simulink model "telegraph"  (R2015b)
settings: Solver=FixedStepAuto  StartTime=0.0  StopTime=50  FixedStep=0.1  RelTol=1e-3
libraries: robotlib x18, dspsrcs4 x6
settings Model: Creator=erik  LastModifiedBy=rasrack
settings OptimizationCC: OptimizeModelRefInitCode=on  LifeSpan=1  MaxStackSize=64
settings HardwareCC: ProdBitPerPointer=32  ProdLargestAtomicFloat=None  ProdIntDivRoundTo=Undefined  ProdEndianess=Unspecified  ProdWordSize=32  ProdHWDeviceType=Generic->Unspecified (assume 32-bit Generic)
settings RTWCC: SystemTargetFile=ert.tlc  TemplateMakefile=ert_default_tmf  Description=Embedded Coder  Toolchain=Catkin  TargetLang=C++
settings CodeAppCC: IgnoreCustomStorageClasses=off
settings ERTTargetCC: GenerateSampleERTMain=on

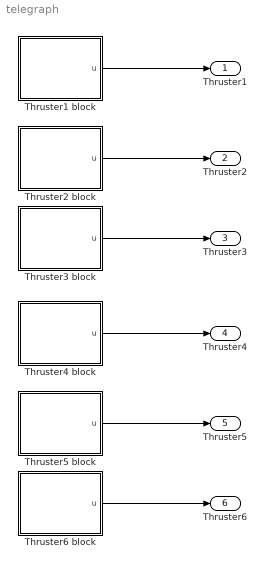
== system telegraph ==
  Thruster1 block : Subsystem
  Thruster2 block : Subsystem
  Thruster3 block : Subsystem
  Thruster4 block : Subsystem
  Thruster5 block : Subsystem
  Thruster6 block : Subsystem
  Thruster1 : Outport
  Thruster2 : Outport  Port=2
  Thruster3 : Outport  Port=3
  Thruster4 : Outport  Port=4
  Thruster5 : Outport  Port=5
  Thruster6 : Outport  Port=6
  wires:
  Thruster1 block/1(u) -> Thruster1/1
  Thruster2 block/1(u) -> Thruster2/1
  Thruster3 block/1(u) -> Thruster3/1
  Thruster4 block/1(u) -> Thruster4/1
  Thruster5 block/1("u ") -> Thruster5/1
  Thruster6 block/1(u) -> Thruster6/1

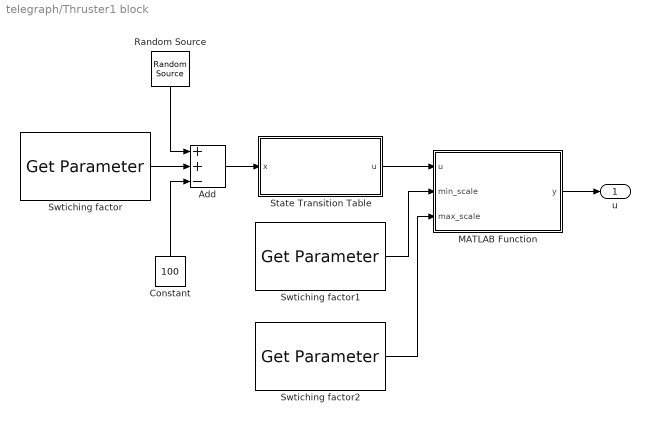
== system telegraph/Thruster1 block ==
  Add : Sum  Inputs=++-
  Constant : Constant  Value=100
  MATLAB Function : MATLAB Function  TreatAsAtomicUnit=on
  Random Source : dspsrcs4/Random Source  SrcType=Uniform  NormMethod=Ziggurat  CltLength=12  MinVal=1  MaxVal=100  MeanVal=0  VarVal=1  RepMode=Not repeatable  rawSeed=1  IsInherit=on  SampMode=Discrete  SampTime=0.1  SampFrame=1  DataType=Double  OutComplex=Real  OutputFrames=off
  State Transition Table : State Transition Table  TreatAsAtomicUnit=on
  Swtiching factor : robotlib/Get Parameter  SourceLibraryInfo=This block requires Robotics System Toolbox  ParameterSource=Specify your own  ParameterName=/matlab_controller/thruster1/switch_factor  ParameterType=int32  ParameterInitialValue=0.0  SampleTime=-1  ShowErrorCodeOutput=off  ModelName=telegraph  BlockId=ParamGet_telegraph_32
  Swtiching factor1 : robotlib/Get Parameter  SourceLibraryInfo=This block requires Robotics System Toolbox  ParameterSource=Specify your own  ParameterName=/matlab_controller/thruster1/min_scale  ParameterType=int32  ParameterInitialValue=1  SampleTime=-1  ShowErrorCodeOutput=off  ModelName=telegraph  BlockId=ParamGet_telegraph_50
  Swtiching factor2 : robotlib/Get Parameter  SourceLibraryInfo=This block requires Robotics System Toolbox  ParameterSource=Specify your own  ParameterName=/matlab_controller/thruster1/max_scale  ParameterType=int32  ParameterInitialValue=1.0  SampleTime=-1  ShowErrorCodeOutput=off  ModelName=telegraph  BlockId=ParamGet_telegraph_51
  u : Outport
  wires:
  MATLAB Function/1(y) -> u/1
  Swtiching factor1/1 -> MATLAB Function/2(min_scale)
  State Transition Table/1(u) -> MATLAB Function/1(u)
  Swtiching factor2/1 -> MATLAB Function/3(max_scale)
  Add/1 -> State Transition Table/1(x)
  Swtiching factor/1 -> Add/2
  Random Source/1 -> Add/1
  Constant/1 -> Add/3

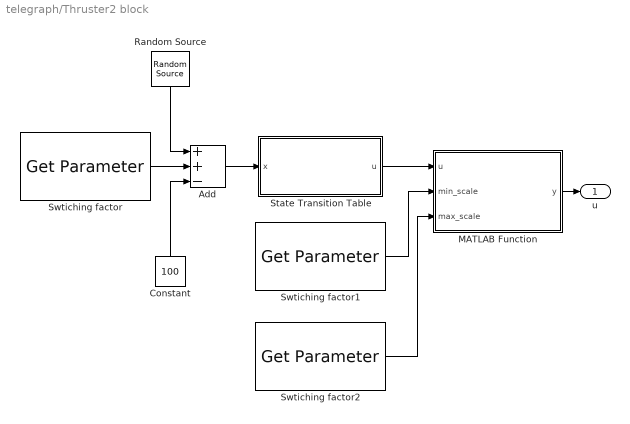
== system telegraph/Thruster2 block ==
  Add : Sum  Inputs=++-
  Constant : Constant  Value=100
  MATLAB Function : MATLAB Function  TreatAsAtomicUnit=on
  Random Source : dspsrcs4/Random Source  SrcType=Uniform  NormMethod=Ziggurat  CltLength=12  MinVal=1  MaxVal=100  MeanVal=0  VarVal=1  RepMode=Not repeatable  rawSeed=1  IsInherit=on  SampMode=Discrete  SampTime=0.1  SampFrame=1  DataType=Double  OutComplex=Real  OutputFrames=off
  State Transition Table : State Transition Table  TreatAsAtomicUnit=on
  Swtiching factor : robotlib/Get Parameter  SourceLibraryInfo=This block requires Robotics System Toolbox  ParameterSource=Specify your own  ParameterName=/matlab_controller/thruster2/switch_factor  ParameterType=int32  ParameterInitialValue=0.0  SampleTime=-1  ShowErrorCodeOutput=off  ModelName=telegraph  BlockId=ParamGet_telegraph_60
  Swtiching factor1 : robotlib/Get Parameter  SourceLibraryInfo=This block requires Robotics System Toolbox  ParameterSource=Specify your own  ParameterName=/matlab_controller/thruster2/min_scale  ParameterType=int32  ParameterInitialValue=1  SampleTime=-1  ShowErrorCodeOutput=off  ModelName=telegraph  BlockId=ParamGet_telegraph_61
  Swtiching factor2 : robotlib/Get Parameter  SourceLibraryInfo=This block requires Robotics System Toolbox  ParameterSource=Specify your own  ParameterName=/matlab_controller/thruster2/max_scale  ParameterType=int32  ParameterInitialValue=1.0  SampleTime=-1  ShowErrorCodeOutput=off  ModelName=telegraph  BlockId=ParamGet_telegraph_62
  u : Outport
  wires:
  MATLAB Function/1(y) -> u/1
  Swtiching factor1/1 -> MATLAB Function/2(min_scale)
  State Transition Table/1(u) -> MATLAB Function/1(u)
  Swtiching factor2/1 -> MATLAB Function/3(max_scale)
  Add/1 -> State Transition Table/1(x)
  Swtiching factor/1 -> Add/2
  Random Source/1 -> Add/1
  Constant/1 -> Add/3

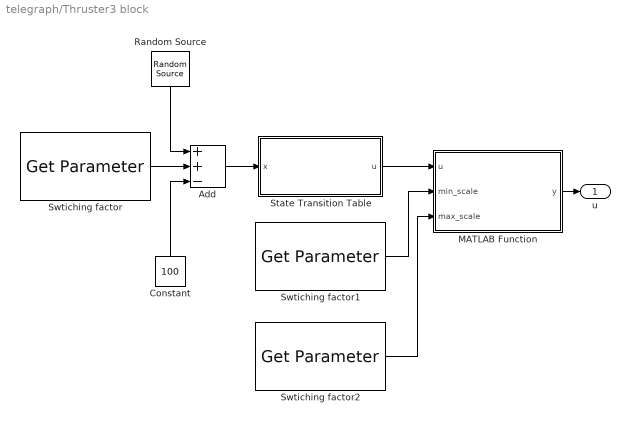
== system telegraph/Thruster3 block ==
  Add : Sum  Inputs=++-
  Constant : Constant  Value=100
  MATLAB Function : MATLAB Function  TreatAsAtomicUnit=on
  Random Source : dspsrcs4/Random Source  SrcType=Uniform  NormMethod=Ziggurat  CltLength=12  MinVal=1  MaxVal=100  MeanVal=0  VarVal=1  RepMode=Not repeatable  rawSeed=1  IsInherit=on  SampMode=Discrete  SampTime=0.1  SampFrame=1  DataType=Double  OutComplex=Real  OutputFrames=off
  State Transition Table : State Transition Table  TreatAsAtomicUnit=on
  Swtiching factor : robotlib/Get Parameter  SourceLibraryInfo=This block requires Robotics System Toolbox  ParameterSource=Specify your own  ParameterName=/matlab_controller/thruster3/switch_factor  ParameterType=int32  ParameterInitialValue=0.0  SampleTime=-1  ShowErrorCodeOutput=off  ModelName=telegraph  BlockId=ParamGet_telegraph_70
  Swtiching factor1 : robotlib/Get Parameter  SourceLibraryInfo=This block requires Robotics System Toolbox  ParameterSource=Specify your own  ParameterName=/matlab_controller/thruster3/min_scale  ParameterType=int32  ParameterInitialValue=1  SampleTime=-1  ShowErrorCodeOutput=off  ModelName=telegraph  BlockId=ParamGet_telegraph_71
  Swtiching factor2 : robotlib/Get Parameter  SourceLibraryInfo=This block requires Robotics System Toolbox  ParameterSource=Specify your own  ParameterName=/matlab_controller/thruster3/max_scale  ParameterType=int32  ParameterInitialValue=1.0  SampleTime=-1  ShowErrorCodeOutput=off  ModelName=telegraph  BlockId=ParamGet_telegraph_72
  u : Outport
  wires:
  MATLAB Function/1(y) -> u/1
  Swtiching factor1/1 -> MATLAB Function/2(min_scale)
  State Transition Table/1(u) -> MATLAB Function/1(u)
  Swtiching factor2/1 -> MATLAB Function/3(max_scale)
  Add/1 -> State Transition Table/1(x)
  Swtiching factor/1 -> Add/2
  Random Source/1 -> Add/1
  Constant/1 -> Add/3

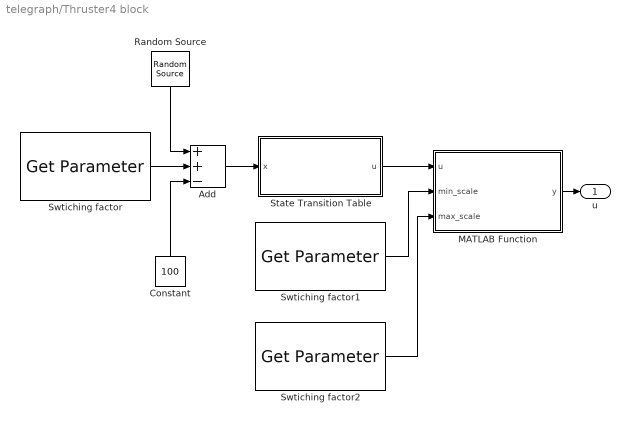
== system telegraph/Thruster4 block ==
  Add : Sum  Inputs=++-
  Constant : Constant  Value=100
  MATLAB Function : MATLAB Function  TreatAsAtomicUnit=on
  Random Source : dspsrcs4/Random Source  SrcType=Uniform  NormMethod=Ziggurat  CltLength=12  MinVal=1  MaxVal=100  MeanVal=0  VarVal=1  RepMode=Not repeatable  rawSeed=1  IsInherit=on  SampMode=Discrete  SampTime=0.1  SampFrame=1  DataType=Double  OutComplex=Real  OutputFrames=off
  State Transition Table : State Transition Table  TreatAsAtomicUnit=on
  Swtiching factor : robotlib/Get Parameter  SourceLibraryInfo=This block requires Robotics System Toolbox  ParameterSource=Specify your own  ParameterName=/matlab_controller/thruster4/switch_factor  ParameterType=int32  ParameterInitialValue=0.0  SampleTime=-1  ShowErrorCodeOutput=off  ModelName=telegraph  BlockId=ParamGet_telegraph_80
  Swtiching factor1 : robotlib/Get Parameter  SourceLibraryInfo=This block requires Robotics System Toolbox  ParameterSource=Specify your own  ParameterName=/matlab_controller/thruster4/min_scale  ParameterType=int32  ParameterInitialValue=1  SampleTime=-1  ShowErrorCodeOutput=off  ModelName=telegraph  BlockId=ParamGet_telegraph_81
  Swtiching factor2 : robotlib/Get Parameter  SourceLibraryInfo=This block requires Robotics System Toolbox  ParameterSource=Specify your own  ParameterName=/matlab_controller/thruster4/max_scale  ParameterType=int32  ParameterInitialValue=1.0  SampleTime=-1  ShowErrorCodeOutput=off  ModelName=telegraph  BlockId=ParamGet_telegraph_82
  u : Outport
  wires:
  MATLAB Function/1(y) -> u/1
  Swtiching factor1/1 -> MATLAB Function/2(min_scale)
  State Transition Table/1(u) -> MATLAB Function/1(u)
  Swtiching factor2/1 -> MATLAB Function/3(max_scale)
  Add/1 -> State Transition Table/1(x)
  Swtiching factor/1 -> Add/2
  Random Source/1 -> Add/1
  Constant/1 -> Add/3

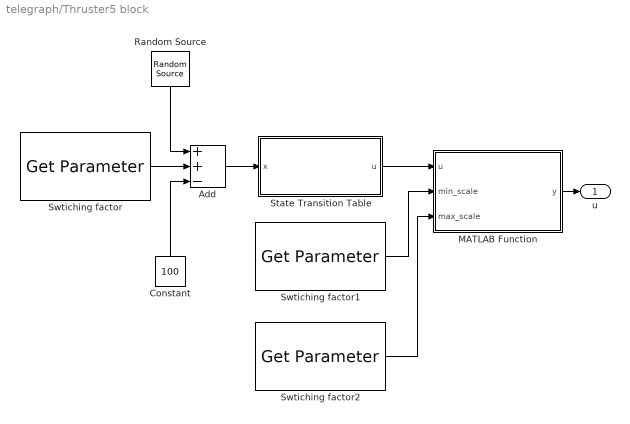
== system telegraph/Thruster5 block ==
  Add : Sum  Inputs=++-
  Constant : Constant  Value=100
  MATLAB Function : MATLAB Function  TreatAsAtomicUnit=on
  Random Source : dspsrcs4/Random Source  SrcType=Uniform  NormMethod=Ziggurat  CltLength=12  MinVal=1  MaxVal=100  MeanVal=0  VarVal=1  RepMode=Not repeatable  rawSeed=1  IsInherit=on  SampMode=Discrete  SampTime=0.1  SampFrame=1  DataType=Double  OutComplex=Real  OutputFrames=off
  State Transition Table : State Transition Table  TreatAsAtomicUnit=on
  Swtiching factor : robotlib/Get Parameter  SourceLibraryInfo=This block requires Robotics System Toolbox  ParameterSource=Specify your own  ParameterName=/matlab_controller/thruster5/switch_factor  ParameterType=int32  ParameterInitialValue=0.0  SampleTime=-1  ShowErrorCodeOutput=off  ModelName=telegraph  BlockId=ParamGet_telegraph_90
  Swtiching factor1 : robotlib/Get Parameter  SourceLibraryInfo=This block requires Robotics System Toolbox  ParameterSource=Specify your own  ParameterName=/matlab_controller/thruster5/min_scale  ParameterType=int32  ParameterInitialValue=1  SampleTime=-1  ShowErrorCodeOutput=off  ModelName=telegraph  BlockId=ParamGet_telegraph_91
  Swtiching factor2 : robotlib/Get Parameter  SourceLibraryInfo=This block requires Robotics System Toolbox  ParameterSource=Specify your own  ParameterName=/matlab_controller/thruster5/max_scale  ParameterType=int32  ParameterInitialValue=1.0  SampleTime=-1  ShowErrorCodeOutput=off  ModelName=telegraph  BlockId=ParamGet_telegraph_92
  "u " : Outport
  wires:
  MATLAB Function/1(y) -> "u "/1
  Swtiching factor1/1 -> MATLAB Function/2(min_scale)
  State Transition Table/1(u) -> MATLAB Function/1(u)
  Swtiching factor2/1 -> MATLAB Function/3(max_scale)
  Add/1 -> State Transition Table/1(x)
  Swtiching factor/1 -> Add/2
  Random Source/1 -> Add/1
  Constant/1 -> Add/3

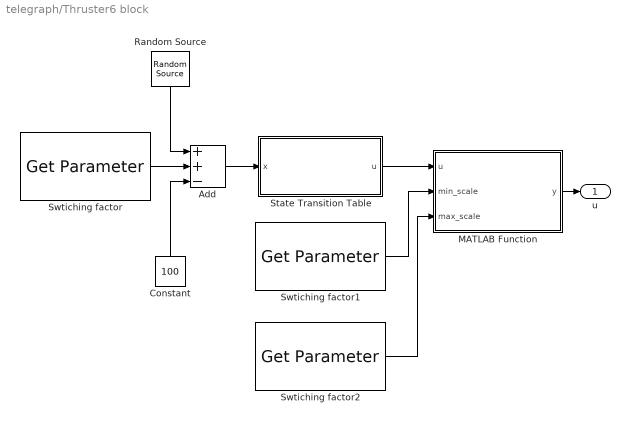
== system telegraph/Thruster6 block ==
  Add : Sum  Inputs=++-
  Constant : Constant  Value=100
  MATLAB Function : MATLAB Function  TreatAsAtomicUnit=on
  Random Source : dspsrcs4/Random Source  SrcType=Uniform  NormMethod=Ziggurat  CltLength=12  MinVal=1  MaxVal=100  MeanVal=0  VarVal=1  RepMode=Not repeatable  rawSeed=1  IsInherit=on  SampMode=Discrete  SampTime=0.1  SampFrame=1  DataType=Double  OutComplex=Real  OutputFrames=off
  State Transition Table : State Transition Table  TreatAsAtomicUnit=on
  Swtiching factor : robotlib/Get Parameter  SourceLibraryInfo=This block requires Robotics System Toolbox  ParameterSource=Specify your own  ParameterName=/matlab_controller/thruster6/switch_factor  ParameterType=int32  ParameterInitialValue=0.0  SampleTime=-1  ShowErrorCodeOutput=off  ModelName=telegraph  BlockId=ParamGet_telegraph_100
  Swtiching factor1 : robotlib/Get Parameter  SourceLibraryInfo=This block requires Robotics System Toolbox  ParameterSource=Specify your own  ParameterName=/matlab_controller/thruster6/min_scale  ParameterType=int32  ParameterInitialValue=1  SampleTime=-1  ShowErrorCodeOutput=off  ModelName=telegraph  BlockId=ParamGet_telegraph_101
  Swtiching factor2 : robotlib/Get Parameter  SourceLibraryInfo=This block requires Robotics System Toolbox  ParameterSource=Specify your own  ParameterName=/matlab_controller/thruster6/max_scale  ParameterType=int32  ParameterInitialValue=1.0  SampleTime=-1  ShowErrorCodeOutput=off  ModelName=telegraph  BlockId=ParamGet_telegraph_102
  u : Outport
  wires:
  MATLAB Function/1(y) -> u/1
  Swtiching factor1/1 -> MATLAB Function/2(min_scale)
  State Transition Table/1(u) -> MATLAB Function/1(u)
  Swtiching factor2/1 -> MATLAB Function/3(max_scale)
  Add/1 -> State Transition Table/1(x)
  Swtiching factor/1 -> Add/2
  Random Source/1 -> Add/1
  Constant/1 -> Add/3

== matlab function telegraph/Thruster2 block/MATLAB Function ==
  data: u input; y output; min_scale input; max_scale input
function y = fcn(u,min_scale,max_scale)
%#codegen
    
    if (u < 0)
        y = min_scale*u;
    else
        y = max_scale*u;
    end
end

== matlab function telegraph/Thruster1 block/MATLAB Function ==
  data: u input; y output; min_scale input; max_scale input
function y = fcn(u,min_scale,max_scale)
%#codegen
    
    if (u < 0)
        y = min_scale*u;
    else
        y = max_scale*u;
    end
end

== stateflow chart telegraph/Thruster2 block/State Transition Table ==
  state state1
  state state2
  (default) -> state1
  state1 -> (junction 20) [order 2]
  (junction 20) -> state1
  state1 -> state2 [order 1] : [x > 0]
      | {u = 1}
  state2 -> state1 [order 1] : [x> 0]
      | {u= -1}
  state2 -> (junction 24) [order 2]
  (junction 24) -> state2
  data: x input; u output

== stateflow chart telegraph/Thruster1 block/State Transition Table ==
  state state1
  state state2
  (default) -> state1
  state1 -> (junction 20) [order 2]
  (junction 20) -> state1
  state1 -> state2 [order 1] : [x > 0]
      | {u = 1}
  state2 -> state1 [order 1] : [x> 0]
      | {u= -1}
  state2 -> (junction 24) [order 2]
  (junction 24) -> state2
  data: x input; u output

== matlab function telegraph/Thruster3 block/MATLAB Function ==
  data: u input; y output; min_scale input; max_scale input
function y = fcn(u,min_scale,max_scale)
%#codegen
    
    if (u < 0)
        y = min_scale*u;
    else
        y = max_scale*u;
    end
end

== stateflow chart telegraph/Thruster3 block/State Transition Table ==
  state state1
  state state2
  (default) -> state1
  state1 -> (junction 20) [order 2]
  (junction 20) -> state1
  state1 -> state2 [order 1] : [x > 0]
      | {u = 1}
  state2 -> state1 [order 1] : [x> 0]
      | {u= -1}
  state2 -> (junction 24) [order 2]
  (junction 24) -> state2
  data: x input; u output

== matlab function telegraph/Thruster4 block/MATLAB Function ==
  data: u input; y output; min_scale input; max_scale input
function y = fcn(u,min_scale,max_scale)
%#codegen
    
    if (u < 0)
        y = min_scale*u;
    else
        y = max_scale*u;
    end
end

== stateflow chart telegraph/Thruster4 block/State Transition Table ==
  state state1
  state state2
  (default) -> state1
  state1 -> (junction 20) [order 2]
  (junction 20) -> state1
  state1 -> state2 [order 1] : [x > 0]
      | {u = 1}
  state2 -> state1 [order 1] : [x> 0]
      | {u= -1}
  state2 -> (junction 24) [order 2]
  (junction 24) -> state2
  data: x input; u output

== matlab function telegraph/Thruster5 block/MATLAB Function ==
  data: u input; y output; min_scale input; max_scale input
function y = fcn(u,min_scale,max_scale)
%#codegen
    
    if (u < 0)
        y = min_scale*u;
    else
        y = max_scale*u;
    end
end

== stateflow chart telegraph/Thruster5 block/State Transition Table ==
  state state1
  state state2
  (default) -> state1
  state1 -> (junction 20) [order 2]
  (junction 20) -> state1
  state1 -> state2 [order 1] : [x > 0]
      | {u = 1}
  state2 -> state1 [order 1] : [x> 0]
      | {u= -1}
  state2 -> (junction 24) [order 2]
  (junction 24) -> state2
  data: x input; u output

== matlab function telegraph/Thruster6 block/MATLAB Function ==
  data: u input; y output; min_scale input; max_scale input
function y = fcn(u,min_scale,max_scale)
%#codegen
    
    if (u < 0)
        y = min_scale*u;
    else
        y = max_scale*u;
    end
end

== stateflow chart telegraph/Thruster6 block/State Transition Table ==
  state state1
  state state2
  (default) -> state1
  state1 -> (junction 20) [order 2]
  (junction 20) -> state1
  state1 -> state2 [order 1] : [x > 0]
      | {u = 1}
  state2 -> state1 [order 1] : [x> 0]
      | {u= -1}
  state2 -> (junction 24) [order 2]
  (junction 24) -> state2
  data: x input; u output
